simulink model "sysgenTripleBuffer"  (Simulink 7.7)
settings: Solver=ode3  SolverMode=SingleTasking  StartTime=0.0  StopTime=inf  FixedStep=1  RelTol=1e-3
PreLoadFcn:
  | sysgenTripleBuffer_PreloadFcn
undefined symbols (not defined in the file or in its folder): c_hsync, c_image_cols, c_image_rows, c_vsync, c_word_size, gray, pixel_period, videoFrame
libraries: xbsIndex_r4 x101, simulink x4, dspsigattribs x3, dspbuff3 x3, dspmtrx3 x3, xbsCopyrightNotice_r4 x1, vipsnks x1, vipsrcs x1
(part 2 of 2)

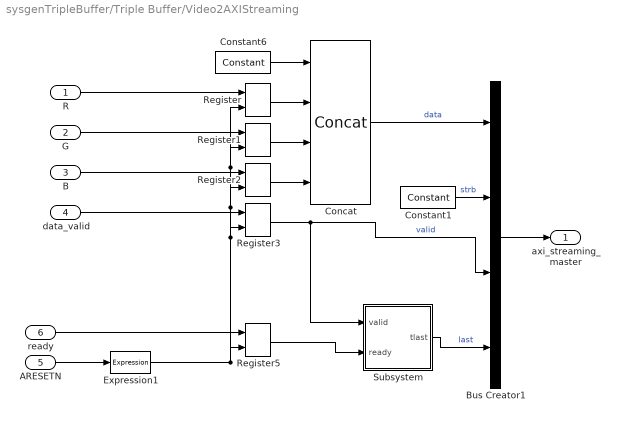
== system sysgenTripleBuffer/Triple Buffer/Video2AXIStreaming ==
  R : Inport
  G : Inport  Port=2
  B : Inport  Port=3
  data_valid : Inport  Port=4
  ARESETN : Inport  Port=5
  ready : Inport  Port=6
  Bus Creator1 : BusCreator
  Concat : xbsIndex_r4/Concat  num_inputs=4  dbl_ovrd=off  block_type=concat
      settings: block_version=12.3
  Constant1 : xbsIndex_r4/Constant  const=2^4-1  gui_display_data_type=Fixed-point  arith_type=Unsigned  n_bits=4  bin_pt=0  preci_type=Single  exp_width=8  frac_width=24  explicit_period=on  period=pixel_period  equ=P=C  opselect=C  inp2=PCIN>>17  opr=+  inp1=P  carry=CIN  dbl_ovrd=off  block_type=constant
      settings: block_version=12.3
  Constant6 : xbsIndex_r4/Constant  const=0  gui_display_data_type=Fixed-point  arith_type=Unsigned  n_bits=8  bin_pt=0  preci_type=Single  exp_width=8  frac_width=24  explicit_period=on  period=pixel_period  equ=P=C  opselect=C  inp2=PCIN>>17  opr=+  inp1=P  carry=CIN  dbl_ovrd=off  block_type=constant
      settings: block_version=12.3
  Expression1 : xbsIndex_r4/Expression  expression=~a  align_bp=on  en=off  latency=0  precision=Full  arith_type=Unsigned  n_bits=16  bin_pt=0  dbl_ovrd=off  block_type=expr
      settings: block_version=13.4
  Register{,1..3,5} (5 alike) : xbsIndex_r4/Register  init=0  rst=on  en=off  dbl_ovrd=off  block_type=register
      settings: block_version=12.3
  Subsystem : Subsystem
  axi_streaming_master : Outport
  wires:
  Constant6/1 -> Concat/1
  Register/1 -> Concat/2
  Register1/1 -> Concat/3
  Register2/1 -> Concat/4
  Register3/1 -> Bus Creator1/3, Subsystem/1(valid)  "valid"
  data_valid/1 -> Register3/1
  ARESETN/1 -> Expression1/1
  Constant1/1 -> Bus Creator1/2  "strb"
  Concat/1 -> Bus Creator1/1  "data"
  Bus Creator1/1 -> axi_streaming_master/1
  Expression1/1 -> Register5/2, Register3/2, Register2/2, Register1/2, Register/2
  Subsystem/1(tlast) -> Bus Creator1/4  "last"
  ready/1 -> Register5/1
  Register5/1 -> Subsystem/2(ready)
  R/1 -> Register/1
  G/1 -> Register1/1
  B/1 -> Register2/1

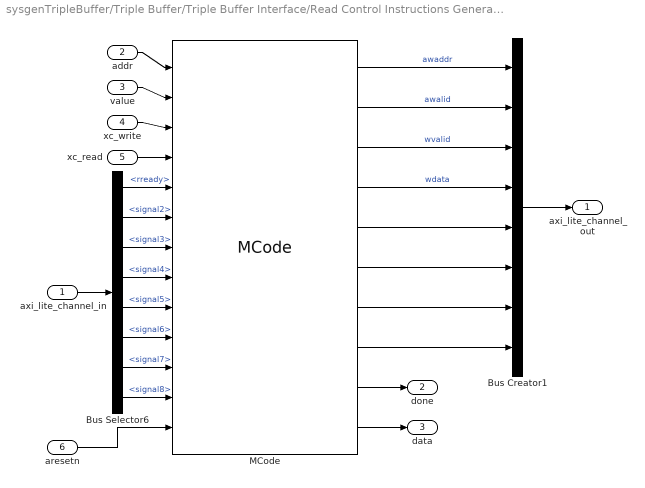
== system sysgenTripleBuffer/Triple Buffer/Triple Buffer Interface/Read Control Instructions Generator1 ==
  axi_lite_channel_in : Inport
  addr : Inport  Port=2
  value : Inport  Port=3
  xc_write : Inport  Port=4
  xc_read : Inport  Port=5
  aresetn : Inport  Port=6
  Bus Creator1 : BusCreator  Inputs=8
  Bus Selector6 : BusSelector  OutputSignals=rready,signal2,signal3,signal4,signal5,signal6,signal7,signal8
  MCode : xbsIndex_r4/MCode  mfname=xlAXILiteVDMACommandDriver  explicit_period=off  period=1  inputsTable={'boundInpExpr'=>['','','','','','','','','','','','',''],'inputs'=>['addr','value','xc_write','xc_read','awready','wready','bresp','bvalid','arready','rvalid','rdata','rresp','aresetn']}  outputsTable={'outputs'=>['awvalid','awaddr','wvalid','wdata','bready','arvalid','araddr','rready','done','read_value'],'suppressOut'=>['off','off','off','off','off','off','off','off','off','off']}  dbl_ovrd=off  enable_stdout=off  enable_debug=off  suppress_output=on  defparams={}  hide_port_list={}  block_type=mcode
      settings: block_version=12.3
  axi_lite_channel_out : Outport
  done : Outport  Port=2
  data : Outport  Port=3
  wires:
  aresetn/1 -> MCode/13
  MCode/10 -> data/1
  xc_write/1 -> MCode/3
  value/1 -> MCode/2
  MCode/9 -> done/1
  xc_read/1 -> MCode/4
  addr/1 -> MCode/1
  MCode/8 -> Bus Creator1/8
  MCode/7 -> Bus Creator1/7
  MCode/6 -> Bus Creator1/6
  MCode/5 -> Bus Creator1/5
  MCode/4 -> Bus Creator1/4  "wdata"
  MCode/3 -> Bus Creator1/3  "wvalid"
  MCode/2 -> Bus Creator1/2  "awalid"
  MCode/1 -> Bus Creator1/1  "awaddr"
  Bus Creator1/1 -> axi_lite_channel_out/1
  axi_lite_channel_in/1 -> Bus Selector6/1
  Bus Selector6/8 -> MCode/12  "<signal8>"
  Bus Selector6/7 -> MCode/11  "<signal7>"
  Bus Selector6/6 -> MCode/10  "<signal6>"
  Bus Selector6/5 -> MCode/9  "<signal5>"
  Bus Selector6/4 -> MCode/8  "<signal4>"
  Bus Selector6/3 -> MCode/7  "<signal3>"
  Bus Selector6/2 -> MCode/6  "<signal2>"
  Bus Selector6/1 -> MCode/5  "<rready>"

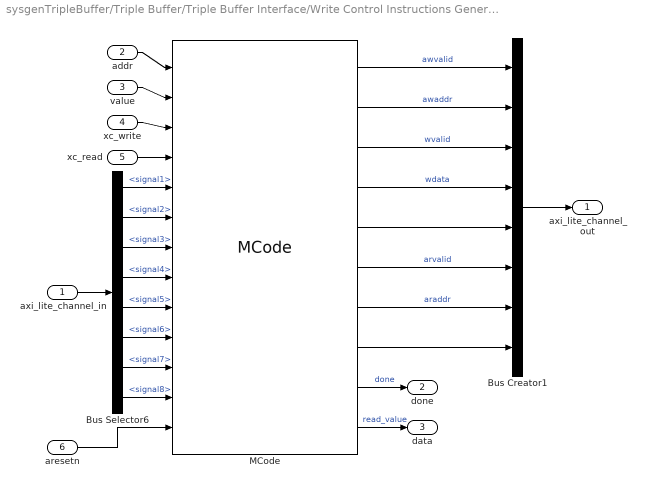
== system sysgenTripleBuffer/Triple Buffer/Triple Buffer Interface/Write Control Instructions Generator ==
  axi_lite_channel_in : Inport
  addr : Inport  Port=2
  value : Inport  Port=3
  xc_write : Inport  Port=4
  xc_read : Inport  Port=5
  aresetn : Inport  Port=6
  Bus Creator1 : BusCreator  Inputs=8
  Bus Selector6 : BusSelector  OutputSignals=signal1,signal2,signal3,signal4,signal5,signal6,signal7,signal8
  MCode : xbsIndex_r4/MCode  mfname=xlAXILiteVDMACommandDriver  explicit_period=off  period=1  inputsTable={'boundInpExpr'=>['','','','','','','','','','','','',''],'inputs'=>['addr','value','xc_write','xc_read','awready','wready','bresp','bvalid','arready','rvalid','rdata','rresp','aresetn']}  outputsTable={'outputs'=>['awvalid','awaddr','wvalid','wdata','bready','arvalid','araddr','rready','done','read_value'],'suppressOut'=>['off','off','off','off','off','off','off','off','off','off']}  dbl_ovrd=off  enable_stdout=off  enable_debug=off  suppress_output=on  defparams={}  hide_port_list={}  block_type=mcode
      settings: block_version=12.3
  axi_lite_channel_out : Outport
  done : Outport  Port=2
  data : Outport  Port=3
  wires:
  Bus Selector6/1 -> MCode/5  "<signal1>"
  Bus Selector6/2 -> MCode/6  "<signal2>"
  Bus Selector6/3 -> MCode/7  "<signal3>"
  Bus Selector6/4 -> MCode/8  "<signal4>"
  Bus Selector6/5 -> MCode/9  "<signal5>"
  Bus Selector6/6 -> MCode/10  "<signal6>"
  Bus Selector6/7 -> MCode/11  "<signal7>"
  Bus Selector6/8 -> MCode/12  "<signal8>"
  axi_lite_channel_in/1 -> Bus Selector6/1
  Bus Creator1/1 -> axi_lite_channel_out/1
  MCode/1 -> Bus Creator1/1  "awvalid"
  MCode/2 -> Bus Creator1/2  "awaddr"
  MCode/3 -> Bus Creator1/3  "wvalid"
  MCode/4 -> Bus Creator1/4  "wdata"
  MCode/5 -> Bus Creator1/5
  MCode/6 -> Bus Creator1/6  "arvalid"
  MCode/7 -> Bus Creator1/7  "araddr"
  MCode/8 -> Bus Creator1/8
  addr/1 -> MCode/1
  xc_read/1 -> MCode/4
  MCode/9 -> done/1  "done"
  value/1 -> MCode/2
  xc_write/1 -> MCode/3
  MCode/10 -> data/1  "read_value"
  aresetn/1 -> MCode/13

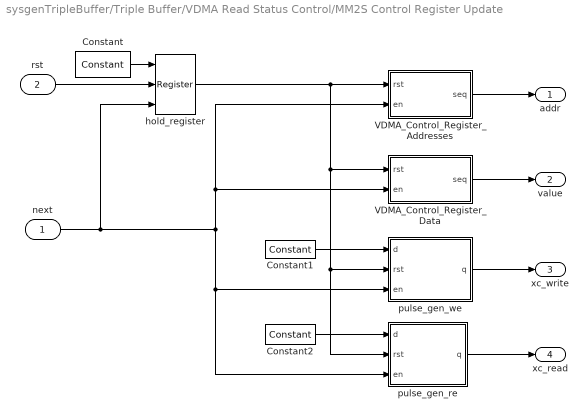
== system sysgenTripleBuffer/Triple Buffer/VDMA Read Status Control/MM2S Control Register Update ==
  next : Inport
  rst : Inport  Port=2
  Constant : xbsIndex_r4/Constant  const=0  gui_display_data_type=Fixed-point  arith_type=Boolean  n_bits=16  bin_pt=14  preci_type=Single  exp_width=8  frac_width=24  explicit_period=on  period=pixel_period  equ=P=C  opselect=C  inp2=PCIN>>17  opr=+  inp1=P  carry=CIN  dbl_ovrd=off  block_type=constant
      settings: block_version=12.3
  Constant1 : xbsIndex_r4/Constant  const=0  gui_display_data_type=Fixed-point  arith_type=Boolean  n_bits=32  bin_pt=0  preci_type=Single  exp_width=8  frac_width=24  explicit_period=on  period=pixel_period  equ=P=C  opselect=C  inp2=PCIN>>17  opr=+  inp1=P  carry=CIN  dbl_ovrd=off  block_type=constant
      settings: block_version=12.3
  Constant2 : xbsIndex_r4/Constant  const=1  gui_display_data_type=Fixed-point  arith_type=Boolean  n_bits=32  bin_pt=0  preci_type=Single  exp_width=8  frac_width=24  explicit_period=on  period=pixel_period  equ=P=C  opselect=C  inp2=PCIN>>17  opr=+  inp1=P  carry=CIN  dbl_ovrd=off  block_type=constant
      settings: block_version=12.3
  VDMA_Control_Register_Addresses : Subsystem  mask{c_sequence=[hex2dec('4') hex2dec('10') hex2dec('0') hex2dec('8') hex2dec('4')]}
      mask prompts: c_sequence "User sequence"
  VDMA_Control_Register_Data : Subsystem  mask{c_sequence=[hex2dec('00007000') 0 hex2dec(['00011013']) 0 hex2dec('00007000')]}
      mask prompts: c_sequence "User sequence"
  hold_register : xbsIndex_r4/Register  init=1  rst=on  en=on  dbl_ovrd=off  block_type=register
      settings: block_version=12.3
  pulse_gen_re : Subsystem
  pulse_gen_we : Subsystem
  addr : Outport
  value : Outport  Port=2
  xc_write : Outport  Port=3
  xc_read : Outport  Port=4
  wires:
  rst/1 -> hold_register/2
  Constant/1 -> hold_register/1
  hold_register/1 -> pulse_gen_re/2(rst), pulse_gen_we/2(rst), VDMA_Control_Register_Data/1(rst), VDMA_Control_Register_Addresses/1(rst)
  pulse_gen_re/1(q) -> xc_read/1
  Constant2/1 -> pulse_gen_re/1(d)
  Constant1/1 -> pulse_gen_we/1(d)
  pulse_gen_we/1(q) -> xc_write/1
  VDMA_Control_Register_Data/1(seq) -> value/1
  VDMA_Control_Register_Addresses/1(seq) -> addr/1
  next/1 -> hold_register/3, pulse_gen_re/3(en), pulse_gen_we/3(en), VDMA_Control_Register_Data/2(en), VDMA_Control_Register_Addresses/2(en)

== system sysgenTripleBuffer/Triple Buffer/VDMA Read Status Control/rising_edge_detector ==
  in : Inport
  rst : Inport  Port=2
  Expression : xbsIndex_r4/Expression  expression=a & ~b  align_bp=on  en=off  latency=0  precision=Full  arith_type=Unsigned  n_bits=16  bin_pt=0  dbl_ovrd=off  block_type=expr
      settings: block_version=12.3
  Register1 : xbsIndex_r4/Register  init=0  rst=on  en=off  dbl_ovrd=off  block_type=register
      settings: block_version=12.3
  rise : Outport
  wires:
  rst/1 -> Register1/2
  Register1/1 -> Expression/2
  in/1 -> Expression/1, Register1/1
  Expression/1 -> rise/1

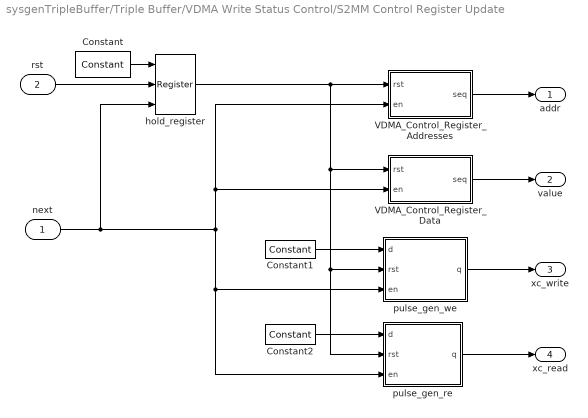
== system sysgenTripleBuffer/Triple Buffer/VDMA Write Status Control/S2MM Control Register Update ==
  next : Inport
  rst : Inport  Port=2
  Constant : xbsIndex_r4/Constant  const=0  gui_display_data_type=Fixed-point  arith_type=Boolean  n_bits=16  bin_pt=14  preci_type=Single  exp_width=8  frac_width=24  explicit_period=on  period=pixel_period  equ=P=C  opselect=C  inp2=PCIN>>17  opr=+  inp1=P  carry=CIN  dbl_ovrd=off  block_type=constant
      settings: block_version=12.3
  Constant1 : xbsIndex_r4/Constant  const=0  gui_display_data_type=Fixed-point  arith_type=Boolean  n_bits=32  bin_pt=0  preci_type=Single  exp_width=8  frac_width=24  explicit_period=on  period=pixel_period  equ=P=C  opselect=C  inp2=PCIN>>17  opr=+  inp1=P  carry=CIN  dbl_ovrd=off  block_type=constant
      settings: block_version=12.3
  Constant2 : xbsIndex_r4/Constant  const=1  gui_display_data_type=Fixed-point  arith_type=Boolean  n_bits=32  bin_pt=0  preci_type=Single  exp_width=8  frac_width=24  explicit_period=on  period=pixel_period  equ=P=C  opselect=C  inp2=PCIN>>17  opr=+  inp1=P  carry=CIN  dbl_ovrd=off  block_type=constant
      settings: block_version=12.3
  VDMA_Control_Register_Addresses : Subsystem  mask{c_sequence=[hex2dec('34') hex2dec('40') hex2dec('30') hex2dec('38') hex2dec('34')]}
      mask prompts: c_sequence "User sequence"
  VDMA_Control_Register_Data : Subsystem  mask{c_sequence=[hex2dec('00007000') 0 hex2dec(['00011013']) 0 hex2dec('00007000')]}
      mask prompts: c_sequence "User sequence"
  hold_register : xbsIndex_r4/Register  init=1  rst=on  en=on  dbl_ovrd=off  block_type=register
      settings: block_version=12.3
  pulse_gen_re : Subsystem
  pulse_gen_we : Subsystem
  addr : Outport
  value : Outport  Port=2
  xc_write : Outport  Port=3
  xc_read : Outport  Port=4
  wires:
  next/1 -> VDMA_Control_Register_Addresses/2(en), VDMA_Control_Register_Data/2(en), pulse_gen_we/3(en), pulse_gen_re/3(en), hold_register/3
  VDMA_Control_Register_Addresses/1(seq) -> addr/1
  VDMA_Control_Register_Data/1(seq) -> value/1
  pulse_gen_we/1(q) -> xc_write/1
  Constant1/1 -> pulse_gen_we/1(d)
  Constant2/1 -> pulse_gen_re/1(d)
  pulse_gen_re/1(q) -> xc_read/1
  hold_register/1 -> pulse_gen_we/2(rst), pulse_gen_re/2(rst), VDMA_Control_Register_Data/1(rst), VDMA_Control_Register_Addresses/1(rst)
  Constant/1 -> hold_register/1
  rst/1 -> hold_register/2

== system sysgenTripleBuffer/Triple Buffer/VDMA Write Status Control/rising_edge_detector ==
  in : Inport
  rst : Inport  Port=2
  Expression : xbsIndex_r4/Expression  expression=a & ~b  align_bp=on  en=off  latency=0  precision=Full  arith_type=Unsigned  n_bits=16  bin_pt=0  dbl_ovrd=off  block_type=expr
      settings: block_version=12.3
  Register1 : xbsIndex_r4/Register  init=0  rst=on  en=off  dbl_ovrd=off  block_type=register
      settings: block_version=12.3
  rise : Outport
  wires:
  rst/1 -> Register1/2
  Register1/1 -> Expression/2
  in/1 -> Expression/1, Register1/1
  Expression/1 -> rise/1

== system sysgenTripleBuffer/Triple Buffer/Video2AXIStreaming/Subsystem ==
  valid : Inport
  ready : Inport  Port=2
  Constant : xbsIndex_r4/Constant  const=c_image_cols-1  gui_display_data_type=Fixed-point  arith_type=Unsigned  n_bits=32  bin_pt=0  preci_type=Single  exp_width=8  frac_width=24  explicit_period=off  period=pixel_period  equ=P=C  opselect=C  inp2=PCIN>>17  opr=+  inp1=P  carry=CIN  dbl_ovrd=off  block_type=constant
      settings: block_version=13.3
  Counter : xbsIndex_r4/Counter  cnt_type=Count Limited  cnt_to=c_image_cols-1  operation=Up  start_count=0  cnt_by_val=1  arith_type=Unsigned  n_bits=32  bin_pt=0  load_pin=off  rst=off  en=on  explicit_period=on  period=pixel_period  dbl_ovrd=off  use_behavioral_HDL=off  implementation=Fabric  block_type=counter
      settings: block_version=13.3
  Logical : xbsIndex_r4/Logical  logical_function=AND  inputs=2  en=off  latency=0  precision=Full  arith_type=Unsigned  n_bits=32  bin_pt=0  align_bp=on  dbl_ovrd=off  block_type=logical
      settings: block_version=13.3
  Relational : xbsIndex_r4/Relational  mode=a=b  en=off  latency=0  dbl_ovrd=off  block_type=relational
      settings: block_version=13.3
  tlast : Outport
  wires:
  Counter/1 -> Relational/1
  Constant/1 -> Relational/2
  Logical/1 -> Counter/1
  valid/1 -> Logical/1
  Relational/1 -> tlast/1
  ready/1 -> Logical/2

== system sysgenTripleBuffer/Triple Buffer/VDMA Read Status Control/MM2S Control Register Update/VDMA_Control_Register_Addresses ==
  rst : Inport
  en : Inport  Port=2
  ROM : xbsIndex_r4/ROM  depth=length(c_sequence)  initVector=c_sequence  distributed_mem=Distributed memory  rst=off  init_reg=0  en=off  latency=0  gui_display_data_type=Fixed-point  arith_type=Unsigned  n_bits=32  bin_pt=0  preci_type=Single  exp_width=8  frac_width=24  dbl_ovrd=off  optimize=Area  use_rpm=on  block_type=sprom
      settings: block_version=12.3
  count_down : Subsystem  mask{init_val=length(c_sequence)-1}
      mask prompts: init_val "Initial Value"
  seq : Outport
  wires:
  en/1 -> count_down/2(en)
  ROM/1 -> seq/1
  rst/1 -> count_down/1(rst)
  count_down/1(cnt) -> ROM/1

== system sysgenTripleBuffer/Triple Buffer/VDMA Read Status Control/MM2S Control Register Update/VDMA_Control_Register_Data ==
  rst : Inport
  en : Inport  Port=2
  ROM : xbsIndex_r4/ROM  depth=length(c_sequence)  initVector=c_sequence  distributed_mem=Distributed memory  rst=off  init_reg=0  en=off  latency=0  gui_display_data_type=Fixed-point  arith_type=Unsigned  n_bits=32  bin_pt=0  preci_type=Single  exp_width=8  frac_width=24  dbl_ovrd=off  optimize=Area  use_rpm=on  block_type=sprom
      settings: block_version=12.3
  count_down : Subsystem  mask{init_val=length(c_sequence)-1}
      mask prompts: init_val "Initial Value"
  seq : Outport
  wires:
  en/1 -> count_down/2(en)
  ROM/1 -> seq/1
  rst/1 -> count_down/1(rst)
  count_down/1(cnt) -> ROM/1

== system sysgenTripleBuffer/Triple Buffer/VDMA Read Status Control/MM2S Control Register Update/pulse_gen_re ==
  d : Inport
  rst : Inport  Port=2
  en : Inport  Port=3
  Register{,1..3} (4 alike) : xbsIndex_r4/Register  init=0  rst=on  en=on  dbl_ovrd=off  block_type=register
      settings: block_version=12.3
  q : Outport
  wires:
  Register3/1 -> q/1
  Register2/1 -> Register3/1
  Register1/1 -> Register2/1
  Register/1 -> Register1/1
  d/1 -> Register/1
  rst/1 -> Register/2, Register3/2, Register2/2, Register1/2
  en/1 -> Register/3, Register3/3, Register2/3, Register1/3

== system sysgenTripleBuffer/Triple Buffer/VDMA Read Status Control/MM2S Control Register Update/pulse_gen_we ==
  d : Inport
  rst : Inport  Port=2
  en : Inport  Port=3
  Register{,1..3} (4 alike) : xbsIndex_r4/Register  init=1  rst=on  en=on  dbl_ovrd=off  block_type=register
      settings: block_version=12.3
  q : Outport
  wires:
  Register3/1 -> q/1
  Register2/1 -> Register3/1
  en/1 -> Register3/3, Register2/3, Register1/3, Register/3
  rst/1 -> Register3/2, Register2/2, Register1/2, Register/2
  d/1 -> Register/1
  Register/1 -> Register1/1
  Register1/1 -> Register2/1

== system sysgenTripleBuffer/Triple Buffer/VDMA Write Status Control/S2MM Control Register Update/VDMA_Control_Register_Addresses ==
  rst : Inport
  en : Inport  Port=2
  ROM : xbsIndex_r4/ROM  depth=length(c_sequence)  initVector=c_sequence  distributed_mem=Distributed memory  rst=off  init_reg=0  en=off  latency=0  gui_display_data_type=Fixed-point  arith_type=Unsigned  n_bits=32  bin_pt=0  preci_type=Single  exp_width=8  frac_width=24  dbl_ovrd=off  optimize=Area  use_rpm=on  block_type=sprom
      settings: block_version=12.3
  count_down : Subsystem  mask{init_val=length(c_sequence)-1}
      mask prompts: init_val "Initial Value"
  seq : Outport
  wires:
  en/1 -> count_down/2(en)
  ROM/1 -> seq/1
  rst/1 -> count_down/1(rst)
  count_down/1(cnt) -> ROM/1

== system sysgenTripleBuffer/Triple Buffer/VDMA Write Status Control/S2MM Control Register Update/VDMA_Control_Register_Data ==
  rst : Inport
  en : Inport  Port=2
  ROM : xbsIndex_r4/ROM  depth=length(c_sequence)  initVector=c_sequence  distributed_mem=Distributed memory  rst=off  init_reg=0  en=off  latency=0  gui_display_data_type=Fixed-point  arith_type=Unsigned  n_bits=32  bin_pt=0  preci_type=Single  exp_width=8  frac_width=24  dbl_ovrd=off  optimize=Area  use_rpm=on  block_type=sprom
      settings: block_version=12.3
  count_down : Subsystem  mask{init_val=length(c_sequence)-1}
      mask prompts: init_val "Initial Value"
  seq : Outport
  wires:
  en/1 -> count_down/2(en)
  ROM/1 -> seq/1
  rst/1 -> count_down/1(rst)
  count_down/1(cnt) -> ROM/1

== system sysgenTripleBuffer/Triple Buffer/VDMA Write Status Control/S2MM Control Register Update/pulse_gen_re ==
  d : Inport
  rst : Inport  Port=2
  en : Inport  Port=3
  Register{,1..3} (4 alike) : xbsIndex_r4/Register  init=0  rst=on  en=on  dbl_ovrd=off  block_type=register
      settings: block_version=12.3
  q : Outport
  wires:
  en/1 -> Register1/3, Register2/3, Register3/3, Register/3
  rst/1 -> Register1/2, Register2/2, Register3/2, Register/2
  d/1 -> Register/1
  Register/1 -> Register1/1
  Register1/1 -> Register2/1
  Register2/1 -> Register3/1
  Register3/1 -> q/1

== system sysgenTripleBuffer/Triple Buffer/VDMA Write Status Control/S2MM Control Register Update/pulse_gen_we ==
  d : Inport
  rst : Inport  Port=2
  en : Inport  Port=3
  Register{,1..3} (4 alike) : xbsIndex_r4/Register  init=1  rst=on  en=on  dbl_ovrd=off  block_type=register
      settings: block_version=12.3
  q : Outport
  wires:
  Register1/1 -> Register2/1
  Register/1 -> Register1/1
  d/1 -> Register/1
  rst/1 -> Register/2, Register1/2, Register2/2, Register3/2
  en/1 -> Register/3, Register1/3, Register2/3, Register3/3
  Register2/1 -> Register3/1
  Register3/1 -> q/1

== system sysgenTripleBuffer/Triple Buffer/VDMA Read Status Control/MM2S Control Register Update/VDMA_Control_Register_Addresses/count_down ==
  rst : Inport
  en : Inport  Port=2
  Constant3 : xbsIndex_r4/Constant  const=0  gui_display_data_type=Fixed-point  arith_type=Unsigned  n_bits=ceil(log2(init_val + 1))  bin_pt=0  preci_type=Single  exp_width=8  frac_width=24  explicit_period=off  period=1  equ=P=C  opselect=C  inp2=PCIN>>17  opr=+  inp1=P  carry=CIN  dbl_ovrd=off  block_type=constant
      settings: block_version=12.3
  Counter : xbsIndex_r4/Counter  cnt_type=Count Limited  cnt_to=0  operation=Down  start_count=init_val  cnt_by_val=1  arith_type=Unsigned  n_bits=ceil(log2(init_val + 1))  bin_pt=0  load_pin=off  rst=on  en=on  explicit_period=on  period=pixel_period  dbl_ovrd=off  use_behavioral_HDL=off  implementation=Fabric  block_type=counter
      settings: block_version=12.3
  Expression : xbsIndex_r4/Expression  expression=a & b  align_bp=on  en=off  latency=0  precision=Full  arith_type=Unsigned  n_bits=16  bin_pt=0  dbl_ovrd=off  block_type=expr
      settings: block_version=12.3
  Relational1 : xbsIndex_r4/Relational  mode=a!=b  en=off  latency=0  dbl_ovrd=off  block_type=relational
      settings: block_version=12.3
  cnt : Outport
  wires:
  rst/1 -> Counter/1
  Expression/1 -> Counter/2
  Counter/1 -> Relational1/1, cnt/1
  Constant3/1 -> Relational1/2
  Relational1/1 -> Expression/1
  en/1 -> Expression/2

== system sysgenTripleBuffer/Triple Buffer/VDMA Read Status Control/MM2S Control Register Update/VDMA_Control_Register_Data/count_down ==
  rst : Inport
  en : Inport  Port=2
  Constant3 : xbsIndex_r4/Constant  const=0  gui_display_data_type=Fixed-point  arith_type=Unsigned  n_bits=ceil(log2(init_val + 1))  bin_pt=0  preci_type=Single  exp_width=8  frac_width=24  explicit_period=off  period=1  equ=P=C  opselect=C  inp2=PCIN>>17  opr=+  inp1=P  carry=CIN  dbl_ovrd=off  block_type=constant
      settings: block_version=12.3
  Counter : xbsIndex_r4/Counter  cnt_type=Count Limited  cnt_to=0  operation=Down  start_count=init_val  cnt_by_val=1  arith_type=Unsigned  n_bits=ceil(log2(init_val + 1))  bin_pt=0  load_pin=off  rst=on  en=on  explicit_period=on  period=pixel_period  dbl_ovrd=off  use_behavioral_HDL=off  implementation=Fabric  block_type=counter
      settings: block_version=12.3
  Expression : xbsIndex_r4/Expression  expression=a & b  align_bp=on  en=off  latency=0  precision=Full  arith_type=Unsigned  n_bits=16  bin_pt=0  dbl_ovrd=off  block_type=expr
      settings: block_version=12.3
  Relational1 : xbsIndex_r4/Relational  mode=a!=b  en=off  latency=0  dbl_ovrd=off  block_type=relational
      settings: block_version=12.3
  cnt : Outport
  wires:
  rst/1 -> Counter/1
  Expression/1 -> Counter/2
  Counter/1 -> Relational1/1, cnt/1
  Constant3/1 -> Relational1/2
  Relational1/1 -> Expression/1
  en/1 -> Expression/2

== system sysgenTripleBuffer/Triple Buffer/VDMA Write Status Control/S2MM Control Register Update/VDMA_Control_Register_Addresses/count_down ==
  rst : Inport
  en : Inport  Port=2
  Constant3 : xbsIndex_r4/Constant  const=0  gui_display_data_type=Fixed-point  arith_type=Unsigned  n_bits=ceil(log2(init_val + 1))  bin_pt=0  preci_type=Single  exp_width=8  frac_width=24  explicit_period=off  period=1  equ=P=C  opselect=C  inp2=PCIN>>17  opr=+  inp1=P  carry=CIN  dbl_ovrd=off  block_type=constant
      settings: block_version=12.3
  Counter : xbsIndex_r4/Counter  cnt_type=Count Limited  cnt_to=0  operation=Down  start_count=init_val  cnt_by_val=1  arith_type=Unsigned  n_bits=ceil(log2(init_val + 1))  bin_pt=0  load_pin=off  rst=on  en=on  explicit_period=off  period=pixel_period  dbl_ovrd=off  use_behavioral_HDL=off  implementation=Fabric  block_type=counter
      settings: block_version=12.3
  Expression : xbsIndex_r4/Expression  expression=a & b  align_bp=on  en=off  latency=0  precision=Full  arith_type=Unsigned  n_bits=16  bin_pt=0  dbl_ovrd=off  block_type=expr
      settings: block_version=12.3
  Relational1 : xbsIndex_r4/Relational  mode=a!=b  en=off  latency=0  dbl_ovrd=off  block_type=relational
      settings: block_version=12.3
  cnt : Outport
  wires:
  rst/1 -> Counter/1
  Expression/1 -> Counter/2
  Counter/1 -> Relational1/1, cnt/1
  Constant3/1 -> Relational1/2
  Relational1/1 -> Expression/1
  en/1 -> Expression/2

== system sysgenTripleBuffer/Triple Buffer/VDMA Write Status Control/S2MM Control Register Update/VDMA_Control_Register_Data/count_down ==
  rst : Inport
  en : Inport  Port=2
  Constant3 : xbsIndex_r4/Constant  const=0  gui_display_data_type=Fixed-point  arith_type=Unsigned  n_bits=ceil(log2(init_val + 1))  bin_pt=0  preci_type=Single  exp_width=8  frac_width=24  explicit_period=off  period=1  equ=P=C  opselect=C  inp2=PCIN>>17  opr=+  inp1=P  carry=CIN  dbl_ovrd=off  block_type=constant
      settings: block_version=12.3
  Counter : xbsIndex_r4/Counter  cnt_type=Count Limited  cnt_to=0  operation=Down  start_count=init_val  cnt_by_val=1  arith_type=Unsigned  n_bits=ceil(log2(init_val + 1))  bin_pt=0  load_pin=off  rst=on  en=on  explicit_period=on  period=pixel_period  dbl_ovrd=off  use_behavioral_HDL=off  implementation=Fabric  block_type=counter
      settings: block_version=12.3
  Expression : xbsIndex_r4/Expression  expression=a & b  align_bp=on  en=off  latency=0  precision=Full  arith_type=Unsigned  n_bits=16  bin_pt=0  dbl_ovrd=off  block_type=expr
      settings: block_version=12.3
  Relational1 : xbsIndex_r4/Relational  mode=a!=b  en=off  latency=0  dbl_ovrd=off  block_type=relational
      settings: block_version=12.3
  cnt : Outport
  wires:
  rst/1 -> Counter/1
  Expression/1 -> Counter/2
  Counter/1 -> Relational1/1, cnt/1
  Constant3/1 -> Relational1/2
  Relational1/1 -> Expression/1
  en/1 -> Expression/2

== matlab function Display/Embedded MATLAB Function ==
  settings: updateMethod=DISCRETE  sampleTime=pixel_period
  data: valid output double; R input double; imageFrame output double; tready output double; G input double; B input double; tvalid input double; tlast input double; aresetn input double; debug_row output double; im_rows input double; im_cols input double; debug_col output double
function [valid, imageFrame, tready, debug_row, debug_col ] = fcn(R,G,B, tvalid, tlast, aresetn, im_rows, im_cols)

persistent imageFrameInternal;
persistent validInternal;
persistent row;
persistent col;

%Adding tready to allow for puncturing
%Puncturing should be implemented 
%using the tready signal
persistent tready_internal;
if isempty(tready_internal),
    tready_internal = 1;
end;

tready = tready_internal;

if (isempty(imageFrameInternal) || aresetn == 0 ),
    imageFrameInternal = zeros(120,160,3);
    validInternal = false;
    row = 1;
    col = 1;
elseif row == 121,
    imageFrameInternal = zeros(120,160,3);
    validInternal = false;
    row = 1;
    col = 1;
end;

if tvalid == 1,
%     if tready_internal == 1,
        imageFrameInternal(row, col, 1) = R;
        imageFrameInternal(row, col, 2) = G;
        imageFrameInternal(row, col, 3) = B;
        col = col + 1;
        %disp(col);
        if tlast == 1,
            row = row + 1;
            col = 1;
        end;
        if row == 121,
            validInternal = true;
        end;
%         tready_internal = 0;
%     else 
%         tready_internal = 1;
%     end
end;    


imageFrame = uint8(imageFrameInternal);
valid = validInternal;
debug_row = row;
debug_col = col;
